simulink model "model2"  (Simulink 7.8)
settings: Solver=ode45  StartTime=0.0  StopTime=100  RelTol=1e-3
settings Model: Creator=nike  LastModifiedBy=nike

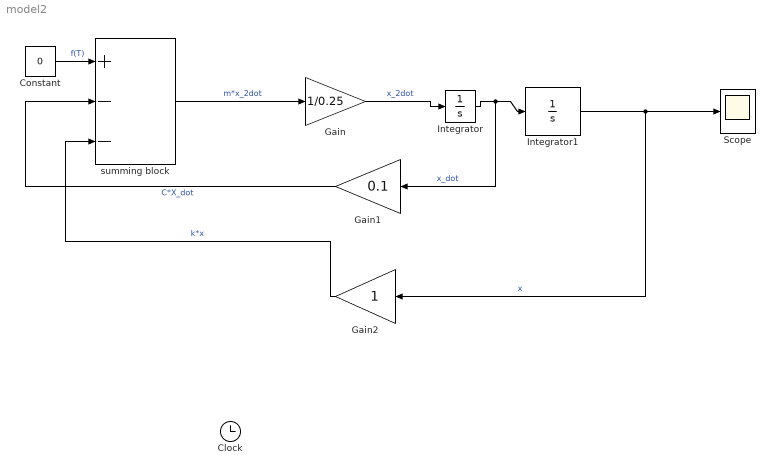
== system model2 ==
  Constant : Constant  Value=0
  Gain : Gain  Gain=1/0.25
  Gain1 : Gain  Gain=0.1
  Gain2 : Gain
  Integrator : Integrator
  Integrator1 : Integrator  InitialCondition=10
  Scope : Scope
      settings: YMax=10
  summing block : Sum  Inputs=+--
  Clock : Clock
      settings: IOType=siggen
  wires:
  Constant/1 -> summing block/1  "f(T)"
  Gain1/1 -> summing block/2  "C*X_dot"
  summing block/1 -> Gain/1  "m*x_2dot"
  Gain/1 -> Integrator/1  "x_2dot"
  Integrator1/1 -> Gain2/1, Scope/1  "x"
  Integrator/1 -> Integrator1/1, Gain1/1  "x_dot"
  Gain2/1 -> summing block/3  "k*x"
